simulink model "Ejercicio_2_d_DB"  (R2023a)
settings: Solver=VariableStepAuto  StartTime=0.0  StopTime=3  RelTol=1e-3
values from neighbouring files (symbols this model uses):
  g0 = utilsMati.realim_VE.factorEscala(A,B,C,K)    [Ejercicio_2_d.m]
  K = acker(A,B,PLC)    [Ejercicio_2_d.m]
settings Model: Creator=Mati  LastModifiedBy=Mati

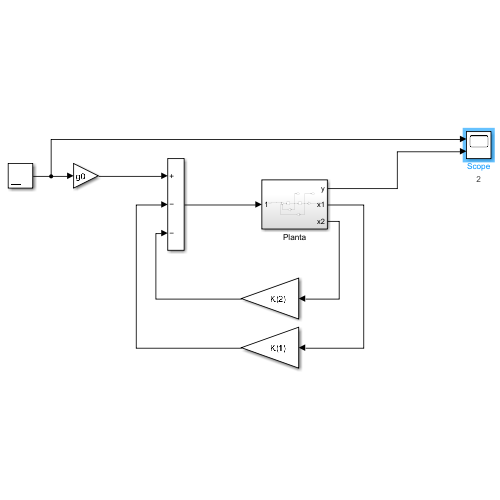
[thumbnail: Simulink's stored preview of the top-level diagram]
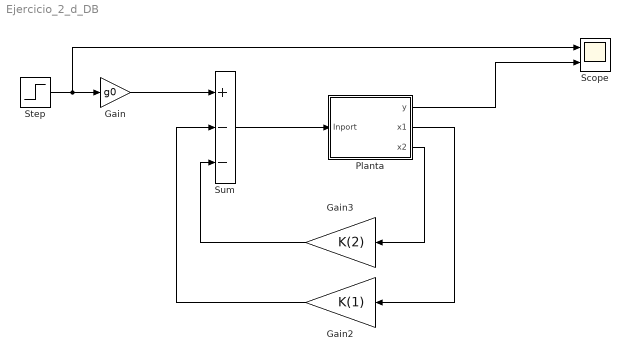
== system Ejercicio_2_d_DB ==
  Gain : Gain  Gain=g0
  Gain2 : Gain  Gain=K(1)
  Gain3 : Gain  Gain=K(2)
  Planta : Subsystem
  Scope : Scope  NumInputPorts=2
      settings: Description=%<NumInputPorts>=2  AttributesFormatString=%<NumInputPorts>
  Step : Step  SampleTime=0
  Sum : Sum  Inputs=+--
  wires:
  Gain/1 -> Sum/1
  Step/1 -> Scope/1, Gain/1
  Sum/1 -> Planta/1(Inport)
  Planta/1(y) -> Scope/2
  Gain2/1 -> Sum/2
  Planta/3(x2) -> Gain3/1
  Planta/2(x1) -> Gain2/1
  Gain3/1 -> Sum/3

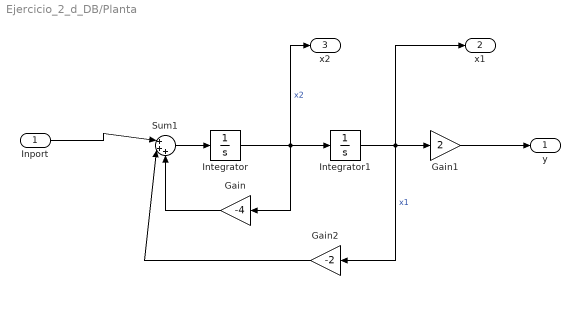
== system Ejercicio_2_d_DB/Planta ==
  Inport : Inport
  Gain : Gain  Gain=-4
  Gain1 : Gain  Gain=2
  Gain2 : Gain  Gain=-2
  Integrator : Integrator
  Integrator1 : Integrator
  Sum1 : Sum  Inputs=|+++
  y : Outport
  x1 : Outport  Port=2
  x2 : Outport  Port=3
  wires:
  Sum1/1 -> Integrator/1
  Inport/1 -> Sum1/1
  Integrator1/1 -> Gain2/1, x1/1, Gain1/1  "x1"
  Integrator/1 -> Gain/1, x2/1, Integrator1/1  "x2"
  Gain1/1 -> y/1
  Gain2/1 -> Sum1/2
  Gain/1 -> Sum1/3
